simulink model "PFMS_Aerosonde_Model"  (Simulink 7.3)
settings: Solver=ode4  SolverMode=SingleTasking  StartTime=0.0  StopTime=inf  FixedStep=0.008  RelTol=1e-3
undefined symbols (not defined in the file or in its folder): b, heading, J, waypoint
libraries: aerosimlib x29, simulink_extras x5
CloseFcn:
  | rtwprivate ssgencode ModelCloseRequest PFMS
settings Model: Creator=Nicholas  LastModifiedBy=user
settings DataIOCC: LimitDataPoints=off  SaveOutput=off  SaveTime=off
settings OptimizationCC: BlockReduction=off  BooleanDataType=off
settings DebuggingCC: SaveWithParameterizedLinksMsg=none  SignalResolutionControl=TryResolveAllWithWarning  SolverPrmCheckMsg=none  MultiTaskDSMMsg=warning  MultiTaskCondExecSysMsg=none  UnconnectedInputMsg=none  UnconnectedOutputMsg=none  UnconnectedLineMsg=none  StrictBusMsg=None
settings HardwareCC: TargetEndianess=LittleEndian  TargetHWDeviceType=MATLAB Host  ProdEqTarget=off
settings RTWCC: IncludeERTFirstTime=on

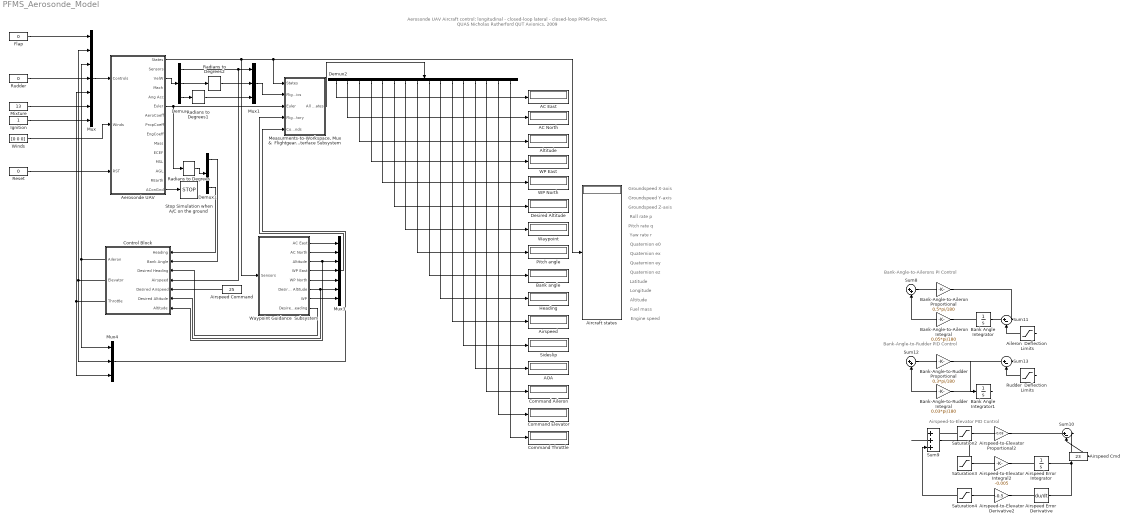
== system PFMS_Aerosonde_Model ==
  note: Groundspeed X-axis
  note: Groundspeed Y-axis
  note: Groundspeed Z-axis
  note: Roll rate p
  note: Pitch rate q
  note: Yaw rate r
  note: Quaternion e0
  note: Quaternion ex
  note: Quaternion ey
  note: Quaternion ez
  note: Latitude
  note: Longitude
  note: Altitude
  note: Fuel mass
  note: Engine speed
  note: Aerosonde UAV
      | Aircraft control: longitudinal - closed-loop
      |   lateral - closed-loop
      | PFMS Project, QUAS
      | Nicholas Rutherford
      | QUT Avionics, 2009
  note: Bank-Angle-to-Ailerons PI Control
  note: Airspeed-to-Elevator PID Control
  note: Bank-Angle-to-Rudder PID Control
  AC East : Display
  AC North : Display
  AOA : Display
  Aerosonde UAV : Subsystem  mask(6-DOF Aircraft Model){aircraftcfg='aerosondecfg.mat', VelocitiesIni=[23 0 0]', RatesIni=[0 0 0]', QuaternionsIni=[1 0 0 0]', PositionIni=[-0.4877  2.6728 1000]', FuelIni=2, OmegaIni=5000*pi/30, GndAlt=20, wmmfile='C:\Program Files\MATLAB\AeroSim\wmm.cof', dmy=[26 05 2009], tsamp=0.8}
      mask prompts: aircraftcfg "Aircraft configuration file:"; VelocitiesIni "Initial velocities:"; RatesIni "Initial angular rates:"; QuaternionsIni "Initial attitude:"; PositionIni "Initial position:"; FuelIni "Initial fuel mass:"; OmegaIni "Initial engine speed:"; GndAlt "Ground altitude:"; wmmfile "WMM coefficient file:"; dmy "Simulation date:"; tsamp "Sample time:"
      mask help: Nonlinear 6-DOF aircraft model with equations of motion in body frame.
      mask init:
      | load(aircraftcfg);
      mask Help:
      | The block implements the 6-DOF nonlinear aircraft model using AeroSim blocks. Velocities are computed in body frame.
      | <P><B>Inputs:</B>
      | <LI>Controls = the 7x1 vector of aircraft controls [flap elevator aileron rudder throttle mixture ignition]. Aerodynamic controls are in radians, throttle is from 0 to 1, mixture is fraction air/fuel flow, ignition is 0 (engine off) or 1 (engine on).</LI>
      | <LI>Winds = the 3x1 vector of background wind speed components in navigation frame [North East Down]</LI>
      | <LI>RST = the integrator reset flag (0 or 1, all integrators on rising edge)
      | </P>
      | <P><B>Outputs:</B>
      | <LI>States = the 15x1 aircraft state vector [Velocities, Angular rates, Quaternions, Position, Fuel mass, Engine speed].</LI>
      | <LI>Sensors = the 18x1 vector of sensor outputs [GPS Position, GPS Groundspeed, Accelerometers, Gyros, Air data, Magnetometer].</LI>
      | <LI>VelW = the 3x1 vector of aircraft velocity in wind axes [Airspeed, sideslip, angle of attack]</LI>
      | <LI>Mach = the Mach number</LI>
      | <LI>Ang Acc = the 3x1 vector of angular accelerations
      | <LI>Euler = the 3x1 vector of Euler angles (roll, pitch, yaw)</LI>
      | <LI>AeroCoeff = the 6x1 vector of aerodynamic coefficients [CD CY CL Cl Cm Cn]</LI>
      | <LI>PropCoeff = the 3x1 vector of propeller coefficients [J CT CP]</LI>
      | <LI>EngCoeff = the 5x1 vector of engine coefficients [MAP Airflow Fuelflow BSFC Power]</LI>
      | <LI>Mass = the current aircraft mass</LI>
      | <LI>ECEF = 3x1 vector of position of the aircraft in the Earth-centered, Earth-fixed frame</LI>
      | <LI>MSL = the aircraft altitude above mean-sea-level</LI>
      | <LI>AGL = the aircraft altitude above terrain</LI>
      | <LI>REarth = the Earth equivalent radius at current location
      | <LI>AConGnd = the aircraft-on-ground flag (0 if aircraft above ground, 1 if aircraft on the ground)</LI>
      | </P>
      | <P><B>Parameters:</B>
      | <LI>Aircraft configuration file = the MAT-file with aircraft data</LI>
      | <LI>Initial velocities = the 3x1 vector of initial aircraft velocities in body axes [u v w]</LI>
      | <LI>Initial angular rates = the 3x1 vector of initial angular rates [p q r]</LI>
      | <LI>Initial attitude = the 4x1 vector of initial quaternions [e0 ex ey ez]</LI>
      | <LI>Initial position = the 3x1 vector of initial aircraft location [Lat Lon Alt]</LI>
      | <LI>Initial fuel mass = the initial quantity of fuel on-board the aircraft</LI>
      | <LI>Initial engine speed = the initial engine rotation speed</LI>
      | <LI>Ground altitude = the ground altitude at aircraft location</LI>
      | <LI>WMM coefficient file = the path to the magnetic model coefficient file</LI>
      | <LI>Simulation date = the date to be used for the magnetic model [day month year]</LI>
      | <LI>Sample time = the aircraft model sample time.</LI>
      | </P>
  Aileron  Deflection  Limits : Saturate  UpperLimit=+20  LowerLimit=-20
  Aircraft states : Display
  Airspeed : Display
  Airspeed Cmd : Constant  Value=23  OutDataType=sfix(16)  OutScaling=2^0
  Airspeed Command : Constant  Value=25
  Airspeed Error Derivative : Derivative
  Airspeed Error Integrator : Integrator
  Airspeed-to-Elevator Derivative2 : Gain  Gain=-0.5  ParameterDataType=sfix(16)  ParameterScaling=2^0  OutDataType=sfix(16)  OutScaling=2^0  SaturateOnIntegerOverflow=on  OutDataTypeStr=Inherit: Same as input  ParamDataTypeStr=Inherit: Same as input
  Airspeed-to-Elevator Integral2 : Gain  Gain=-0.005  ParameterDataType=sfix(16)  ParameterScaling=2^0  OutDataType=sfix(16)  OutScaling=2^0  SaturateOnIntegerOverflow=on  OutDataTypeStr=Inherit: Same as input  ParamDataTypeStr=Inherit: Same as input
  Airspeed-to-Elevator Proportional2 : Gain  Gain=-0.03  ParameterDataType=sfix(16)  ParameterScaling=2^0  OutDataType=sfix(16)  OutScaling=2^0  SaturateOnIntegerOverflow=on  OutDataTypeStr=Inherit: Same as input  ParamDataTypeStr=Inherit: Same as input
  Altitude : Display
  Bank Angle Integrator : Integrator
  Bank Angle Integrator1 : Integrator
  Bank angle : Display
  Bank-Angle-to-Aileron Integral : Gain  Gain=0.05*pi/180  ParameterDataType=sfix(16)  ParameterScaling=2^0  OutDataType=sfix(16)  OutScaling=2^0  SaturateOnIntegerOverflow=on  OutDataTypeStr=Inherit: Same as input  ParamDataTypeStr=Inherit: Same as input
  Bank-Angle-to-Aileron Proportional : Gain  Gain=0.5*pi/180  ParameterDataType=sfix(16)  ParameterScaling=2^0  OutDataType=sfix(16)  OutScaling=2^0  SaturateOnIntegerOverflow=on  OutDataTypeStr=Inherit: Same as input  ParamDataTypeStr=Inherit: Same as input
  Bank-Angle-to-Rudder Integral : Gain  Gain=0.03*pi/180  ParameterDataType=sfix(16)  ParameterScaling=2^0  OutDataType=sfix(16)  OutScaling=2^0  SaturateOnIntegerOverflow=on  OutDataTypeStr=Inherit: Same as input  ParamDataTypeStr=Inherit: Same as input
  Bank-Angle-to-Rudder Proportional : Gain  Gain=0.3*pi/180  ParameterDataType=sfix(16)  ParameterScaling=2^0  OutDataType=sfix(16)  OutScaling=2^0  SaturateOnIntegerOverflow=on  OutDataTypeStr=Inherit: Same as input  ParamDataTypeStr=Inherit: Same as input
  Command Aileron : Display
  Command Elevator : Display
  Command Throttle : Display
  Control Block : Subsystem
  Demux : Demux  Outputs=3
  Demux1 : Demux  Outputs=3
  Demux2 : Demux  Outputs=16
  Desired Altitude : Display
  Flap : Constant  Value=0
  Heading : Display
  Ignition : Constant
  "Measurments-to-Workspace, Mux &  Flightgear Interface Subsystem" : Subsystem
  Mixture : Constant  Value=13
  Mux : Mux  Inputs=7
  Mux1 : Mux  Inputs=3
  Mux3 : Mux  Inputs=7
  Mux4 : Mux  Inputs=3
  Pitch angle : Display
  Radians to Degrees : simulink_extras/Transformations/Radians to Degrees  SystemSampleTime=-1
  Radians to Degrees1 : simulink_extras/Transformations/Radians to Degrees  SystemSampleTime=-1
  Radians to Degrees2 : simulink_extras/Transformations/Radians to Degrees  SystemSampleTime=-1
  Reset : Constant  Value=0
  Rudder : Constant  Value=0
  Rudder  Deflection  Limits : Saturate  UpperLimit=+15  LowerLimit=-15
  Saturation2 : Saturate  UpperLimit=+5  LowerLimit=-5
  Saturation3 : Saturate  UpperLimit=+10  LowerLimit=-10
  Saturation4 : Saturate  UpperLimit=+5  LowerLimit=-5
  Sideslip : Display
  Stop Simulation when A/C on the ground : Stop
  Sum10 : Sum  Inputs=|+-  OutDataType=sfix(16)  OutScaling=2^0  SaturateOnIntegerOverflow=on  InputSameDT=on  OutDataTypeStr=Inherit: Same as first input
  Sum11 : Sum  Inputs=|+-  OutDataType=sfix(16)  OutScaling=2^0  SaturateOnIntegerOverflow=on  InputSameDT=on  OutDataTypeStr=Inherit: Same as first input
  Sum12 : Sum  Inputs=|++  OutDataType=sfix(16)  OutScaling=2^0  SaturateOnIntegerOverflow=on  InputSameDT=on  OutDataTypeStr=Inherit: Same as first input
  Sum13 : Sum  Inputs=|+-  OutDataType=sfix(16)  OutScaling=2^0  SaturateOnIntegerOverflow=on  InputSameDT=on  OutDataTypeStr=Inherit: Same as first input
  Sum8 : Sum  Inputs=|++  OutDataType=sfix(16)  OutScaling=2^0  SaturateOnIntegerOverflow=on  InputSameDT=on  OutDataTypeStr=Inherit: Same as first input
  Sum9 : Sum  Inputs=+++  OutDataType=sfix(16)  OutScaling=2^0  SaturateOnIntegerOverflow=on  InputSameDT=on  OutDataTypeStr=Inherit: Same as first input
  WP East : Display
  WP North : Display
  Waypoint : Display
  Waypoint Guidance  Subsystem : Subsystem
  Winds : Constant  Value=[0 0 0]
  wires:
  Reset/1 -> Aerosonde UAV/3(RST)
  Winds/1 -> Aerosonde UAV/2(Winds)
  Aerosonde UAV/1(States) -> Waypoint Guidance  Subsystem/1(Sensors), Aircraft states/1, "Measurments-to-Workspace, Mux &  Flightgear Interface Subsystem"/1(States)
  Aerosonde UAV/6(Euler) -> Radians to Degrees/1, "Measurments-to-Workspace, Mux &  Flightgear Interface Subsystem"/3(Euler)
  Aerosonde UAV/3(VelW) -> Demux/1
  Demux/3 -> Radians to Degrees1/1
  Demux/2 -> Radians to Degrees2/1
  Demux/1 -> Control Block/4(Airspeed), Mux1/1
  Aerosonde UAV/15(AConGnd) -> Stop Simulation when A/C on the ground/1
  Radians to Degrees/1 -> Demux1/1
  Demux1/1 -> Control Block/2(Bank Angle)
  Rudder/1 -> Mux/4
  Mixture/1 -> Mux/6
  Demux1/3 -> Control Block/1(Heading)
  Airspeed Command/1 -> Control Block/5(Desired Airspeed)
  ? -> Sum13/1, Sum11/1
  Bank-Angle-to-Aileron Proportional/1 -> Sum8/1
  Bank Angle Integrator/1 -> Bank-Angle-to-Aileron Integral/1
  Bank-Angle-to-Aileron Integral/1 -> Sum8/2
  Airspeed Error Derivative/1 -> Airspeed-to-Elevator Derivative2/1
  Airspeed Error Integrator/1 -> Airspeed-to-Elevator Integral2/1
  Airspeed-to-Elevator Proportional2/1 -> Saturation2/1
  Airspeed-to-Elevator Integral2/1 -> Saturation3/1
  Airspeed-to-Elevator Derivative2/1 -> Saturation4/1
  Sum10/1 -> Airspeed-to-Elevator Proportional2/1, Airspeed Error Integrator/1, Airspeed Error Derivative/1
  Sum11/1 -> Bank-Angle-to-Aileron Proportional/1, Bank Angle Integrator/1
  Bank-Angle-to-Rudder Proportional/1 -> Sum12/1
  Bank Angle Integrator1/1 -> Bank-Angle-to-Rudder Integral/1
  Bank-Angle-to-Rudder Integral/1 -> Sum12/2
  Sum13/1 -> Bank-Angle-to-Rudder Proportional/1, Bank Angle Integrator1/1
  Rudder  Deflection  Limits/1 -> Sum13/2
  Aileron  Deflection  Limits/1 -> Sum11/2
  Airspeed Cmd/1 -> Sum10/2
  ? -> Rudder  Deflection  Limits/1, Aileron  Deflection  Limits/1
  Saturation2/1 -> Sum9/1
  Saturation3/1 -> Sum9/2
  Saturation4/1 -> Sum9/3
  ? -> Sum10/1
  Sum8/1 -> ?
  Sum12/1 -> ?
  Sum9/1 -> ?
  Flap/1 -> Mux/1
  Ignition/1 -> Mux/7
  Mux/1 -> Aerosonde UAV/1(Controls)
  Waypoint Guidance  Subsystem/2(AC North) -> Mux3/2
  Waypoint Guidance  Subsystem/4(WP East) -> Mux3/4
  Waypoint Guidance  Subsystem/5(WP North) -> Mux3/5
  Waypoint Guidance  Subsystem/3(Altitude) -> Mux3/3, Control Block/7(Altitude)
  Waypoint Guidance  Subsystem/6(Desired Altitude) -> Mux3/6, Control Block/6(Desired Altitude)
  Waypoint Guidance  Subsystem/8(Desired Heading) -> Control Block/3(Desired Heading)
  Radians to Degrees2/1 -> Mux1/2
  Radians to Degrees1/1 -> Mux1/3
  Mux1/1 -> "Measurments-to-Workspace, Mux &  Flightgear Interface Subsystem"/2(Flight Dynamics)
  Mux3/1 -> "Measurments-to-Workspace, Mux &  Flightgear Interface Subsystem"/4(Flight Trajectory)
  Mux4/1 -> "Measurments-to-Workspace, Mux &  Flightgear Interface Subsystem"/5(Control Commands)
  "Measurments-to-Workspace, Mux &  Flightgear Interface Subsystem"/1(All States) -> Demux2/1
  Waypoint Guidance  Subsystem/7(WP) -> Mux3/7
  Waypoint Guidance  Subsystem/1(AC East) -> Mux3/1
  Control Block/1(Aileron) -> Mux/3, Mux4/1
  Control Block/2(Elevator) -> Mux/2, Mux4/2
  Control Block/3(Throttle) -> Mux4/3, Mux/5
  Demux2/1 -> AC East/1
  Demux2/2 -> AC North/1
  Demux2/3 -> Altitude/1
  Demux2/4 -> WP East/1
  Demux2/5 -> WP North/1
  Demux2/6 -> Desired Altitude/1
  Demux2/7 -> Waypoint/1
  Demux2/8 -> Pitch angle/1
  Demux2/9 -> Bank angle/1
  Demux2/10 -> Heading/1
  Demux2/11 -> Airspeed/1
  Demux2/12 -> Sideslip/1
  Demux2/13 -> AOA/1
  Demux2/14 -> Command Aileron/1
  Demux2/15 -> Command Elevator/1
  Demux2/16 -> Command Throttle/1

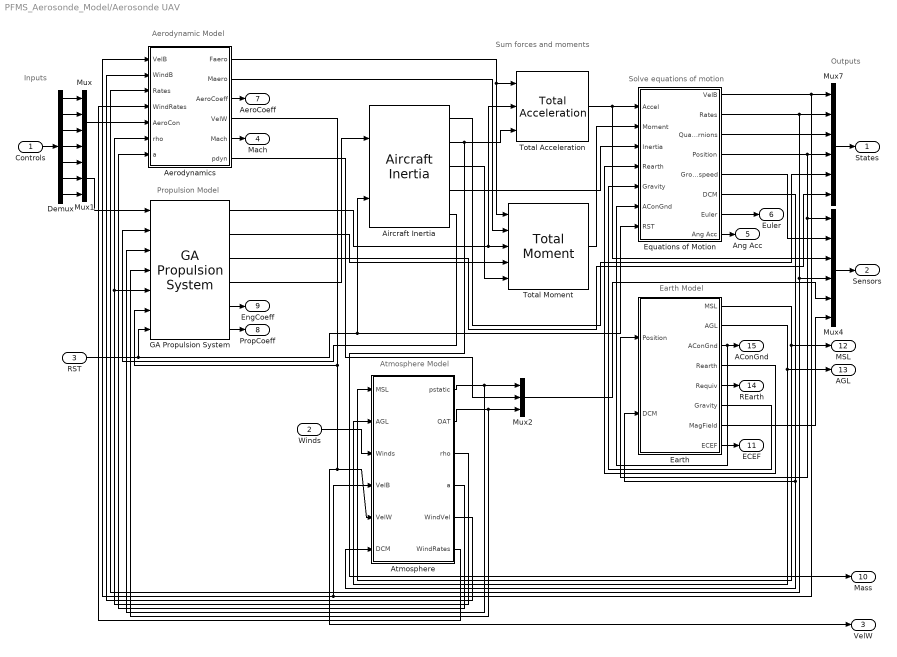
== system PFMS_Aerosonde_Model/Aerosonde UAV ==
  note: Solve equations of motion
  note: Inputs
  note: Outputs
  note: Aerodynamic Model
  note: Earth Model
  note: Sum forces and moments
  note: Atmosphere Model
  note: Propulsion Model
  Controls : Inport  OutDataType=sfix(16)  OutScaling=2^0
  Winds : Inport  Port=2  OutDataType=sfix(16)  OutScaling=2^0
  RST : Inport  Port=3  OutDataType=sfix(16)  OutScaling=2^0
  Aerodynamics : Subsystem
  Aircraft Inertia : aerosimlib/Inertia/Aircraft Inertia  SystemSampleTime=-1  FuelIni=FuelIni  Mempty=mempty  Mgross=mgross  CGempty=CGempty  CGgross=CGgross  Jempty=Jempty  Jgross=Jgross
  Atmosphere : Subsystem
  Demux : Demux  Outputs=7
  Earth : Subsystem
  Equations of Motion : Subsystem
  GA Propulsion System : aerosimlib/Propulsion/GA Propulsion System  SystemSampleTime=-1  OmegaIni=OmegaIni  RPM=RPM  MAP=MAP  FuelFlow=FuelFlow  Power=Power  Jeng=Jeng  J=J  CT=CT  CP=CP  Rprop=Rprop  Jprop=Jprop  TSL=TSL
  Mux : Mux
  Mux1 : Mux  Inputs=3
  Mux2 : Mux  Inputs=3
  Mux4 : Mux  Inputs=6
  Mux7 : Mux  Inputs=6
  Total Acceleration : aerosimlib/Equations of Motion/Total Acceleration  SystemSampleTime=-1
  Total Moment : aerosimlib/Equations of Motion/Total Moment  SystemSampleTime=-1  raero=rAC  rprop=rHub
  States : Outport
  Sensors : Outport  Port=2
  VelW : Outport  Port=3
  Mach : Outport  Port=4
  Ang Acc : Outport  Port=5
  Euler : Outport  Port=6
  AeroCoeff : Outport  Port=7
  PropCoeff : Outport  Port=8
  EngCoeff : Outport  Port=9
  Mass : Outport  Port=10
  ECEF : Outport  Port=11
  MSL : Outport  Port=12
  AGL : Outport  Port=13
  REarth : Outport  Port=14
  AConGnd : Outport  Port=15
  wires:
  Equations of Motion/7(Euler) -> Euler/1
  Equations of Motion/8(Ang Acc) -> Ang Acc/1
  Atmosphere/6(WindRates) -> Aerodynamics/4(WindRates)
  RST/1 -> Aircraft Inertia/2, Equations of Motion/7(RST), GA Propulsion System/7
  Aircraft Inertia/5 -> GA Propulsion System/2
  Atmosphere/4(a) -> Aerodynamics/7(a)
  Atmosphere/3(rho) -> GA Propulsion System/5, Aerodynamics/6(rho)
  Atmosphere/5(WindVel) -> Aerodynamics/2(WindB)
  Winds/1 -> Atmosphere/3(Winds)
  Earth/2(AGL) -> AGL/1, Atmosphere/2(AGL)
  Earth/1(MSL) -> MSL/1, Atmosphere/1(MSL)
  Aerodynamics/4(VelW) -> VelW/1, Atmosphere/5(VelW), GA Propulsion System/6
  GA Propulsion System/4 -> Aircraft Inertia/1
  GA Propulsion System/3 -> Mux7/6
  Aircraft Inertia/1 -> Mux7/5
  Mux2/1 -> Mux4/5
  Aerodynamics/6(pdyn) -> Mux2/2
  Atmosphere/2(OAT) -> GA Propulsion System/4, Mux2/3
  Atmosphere/1(pstatic) -> GA Propulsion System/3, Mux2/1
  Equations of Motion/6(DCM) -> Atmosphere/6(DCM), Earth/2(DCM)
  GA Propulsion System/2 -> Total Moment/4
  GA Propulsion System/1 -> Total Moment/3, Total Acceleration/2
  Aerodynamics/2(Maero) -> Total Moment/2
  Aerodynamics/1(Faero) -> Total Moment/1, Total Acceleration/1
  Aircraft Inertia/3 -> Total Moment/5
  Total Moment/1 -> Equations of Motion/2(Moment)
  Aircraft Inertia/4 -> Equations of Motion/3(Inertia)
  Aircraft Inertia/2 -> Mass/1, Total Acceleration/3
  Earth/4(Rearth) -> Equations of Motion/4(Rearth)
  Earth/6(Gravity) -> Equations of Motion/5(Gravity)
  Earth/7(MagField) -> Mux4/6
  Total Acceleration/1 -> Mux4/3, Equations of Motion/1(Accel)
  Equations of Motion/5(Groundspeed) -> Mux4/2
  Earth/3(AConGnd) -> Equations of Motion/6(AConGnd), AConGnd/1
  Earth/5(Requiv) -> REarth/1
  GA Propulsion System/6 -> PropCoeff/1
  GA Propulsion System/5 -> EngCoeff/1
  Demux/7 -> Mux1/3
  Demux/6 -> Mux1/2
  Demux/5 -> Mux1/1
  Demux/4 -> Mux/4
  Demux/3 -> Mux/3
  Demux/2 -> Mux/2
  Demux/1 -> Mux/1
  Controls/1 -> Demux/1
  Mux4/1 -> Sensors/1
  Mux7/1 -> States/1
  Mux1/1 -> GA Propulsion System/1
  Equations of Motion/1(VelB) -> Aerodynamics/1(VelB), Atmosphere/4(VelB), Mux7/1
  Equations of Motion/2(Rates) -> Aerodynamics/3(Rates), Mux4/4, Mux7/2
  Equations of Motion/4(Position) -> Earth/1(Position), Mux4/1, Mux7/4
  Mux/1 -> Aerodynamics/5(AeroCon)
  Equations of Motion/3(Quaternions) -> Mux7/3
  Aerodynamics/5(Mach) -> Mach/1
  Aerodynamics/3(AeroCoeff) -> AeroCoeff/1
  Earth/8(ECEF) -> ECEF/1

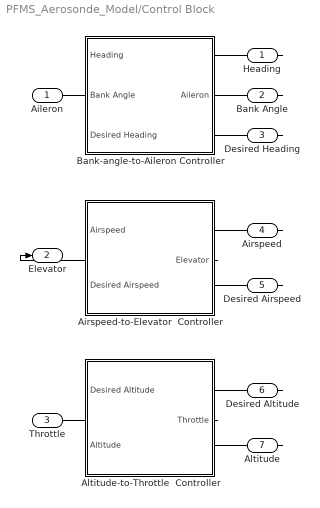
== system PFMS_Aerosonde_Model/Control Block ==
  Heading : Inport
  Bank Angle : Inport  Port=2
  Desired Heading : Inport  Port=3
  Airspeed : Inport  Port=4
  Desired Airspeed : Inport  Port=5
  Desired Altitude : Inport  Port=6
  Altitude : Inport  Port=7
  Airspeed-to-Elevator  Controller : Subsystem
  Altitude-to-Throttle  Controller : Subsystem
  Bank-angle-to-Aileron Controller : Subsystem
  Aileron : Outport
  Elevator : Outport  Port=2
  Throttle : Outport  Port=3
  wires:
  Heading/1 -> Bank-angle-to-Aileron Controller/1(Heading)
  Bank Angle/1 -> Bank-angle-to-Aileron Controller/2(Bank Angle)
  Bank-angle-to-Aileron Controller/1(Aileron) -> Aileron/1
  Desired Heading/1 -> Bank-angle-to-Aileron Controller/3(Desired Heading)
  Airspeed/1 -> Airspeed-to-Elevator  Controller/1(Airspeed)
  Airspeed-to-Elevator  Controller/1(Elevator) -> Elevator/1
  Desired Airspeed/1 -> Airspeed-to-Elevator  Controller/2(Desired Airspeed)
  Desired Altitude/1 -> Altitude-to-Throttle  Controller/1(Desired Altitude)
  Altitude-to-Throttle  Controller/1(Throttle) -> Throttle/1
  Altitude/1 -> Altitude-to-Throttle  Controller/2(Altitude)

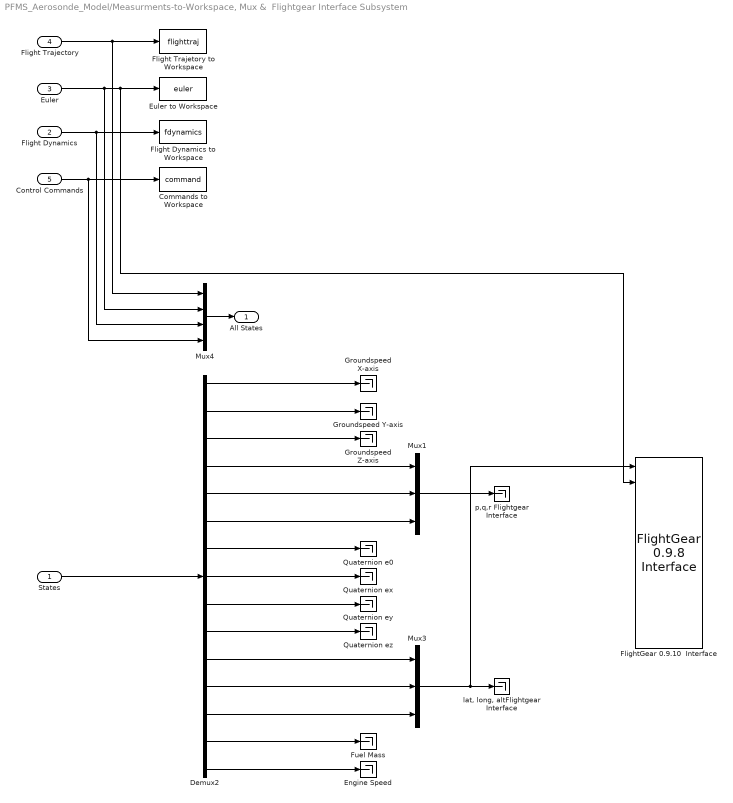
== system PFMS_Aerosonde_Model/Measurments-to-Workspace, Mux &  Flightgear Interface Subsystem ==
  States : Inport
  Flight Dynamics : Inport  Port=2
  Euler : Inport  Port=3
  Flight Trajectory : Inport  Port=4
  Control Commands : Inport  Port=5
  Commands to Workspace : ToWorkspace  VariableName=command  SampleTime=-1  SaveFormat=Structure
  Demux2 : Demux  Outputs=15
  Engine Speed : Terminator
  Euler to Workspace : ToWorkspace  VariableName=euler  SampleTime=-1  SaveFormat=Structure
  Flight Dynamics to Workspace : ToWorkspace  VariableName=fdynamics  SampleTime=-1  SaveFormat=Structure
  Flight Trajetory to Workspace : ToWorkspace  VariableName=flighttraj  SampleTime=-1  SaveFormat=Structure
  FlightGear 0.9.10  Interface : aerosimlib/Pilot Interface/FlightGear 0.9.8  Interface  SystemSampleTime=-1  hostname='localhost'  port=5500  tsamp=0.04
      link override S-Function: FunctionName=sfunflightgear0910
  Fuel Mass : Terminator
  Groundspeed X-axis : Terminator
  Groundspeed Y-axis : Terminator
  Groundspeed Z-axis : Terminator
  Mux1 : Mux  Inputs=3
  Mux3 : Mux  Inputs=3
  Mux4 : Mux
  Quaternion e0 : Terminator
  Quaternion ex : Terminator
  Quaternion ey : Terminator
  Quaternion ez : Terminator
  "lat, long, altFlightgear Interface" : Terminator
  p,q,r Flightgear Interface : Terminator
  All States : Outport  OutDataType=fixdt(1, 16)  OutScaling=2^0
  wires:
  Euler/1 -> Mux4/2, Euler to Workspace/1, FlightGear 0.9.10  Interface/2
  Flight Trajectory/1 -> Flight Trajetory to Workspace/1, Mux4/1
  Flight Dynamics/1 -> Flight Dynamics to Workspace/1, Mux4/3
  Control Commands/1 -> Commands to Workspace/1, Mux4/4
  Mux4/1 -> All States/1
  Demux2/1 -> Groundspeed X-axis/1
  Demux2/2 -> Groundspeed Y-axis/1
  Demux2/3 -> Groundspeed Z-axis/1
  Demux2/4 -> Mux1/1
  Demux2/8 -> Quaternion ex/1
  Demux2/9 -> Quaternion ey/1
  Demux2/10 -> Quaternion ez/1
  Demux2/14 -> Fuel Mass/1
  Demux2/15 -> Engine Speed/1
  Demux2/11 -> Mux3/1
  Demux2/12 -> Mux3/2
  Demux2/13 -> Mux3/3
  States/1 -> Demux2/1
  Demux2/5 -> Mux1/2
  Demux2/6 -> Mux1/3
  Demux2/7 -> Quaternion e0/1
  Mux1/1 -> p,q,r Flightgear Interface/1
  Mux3/1 -> "lat, long, altFlightgear Interface"/1, FlightGear 0.9.10  Interface/1

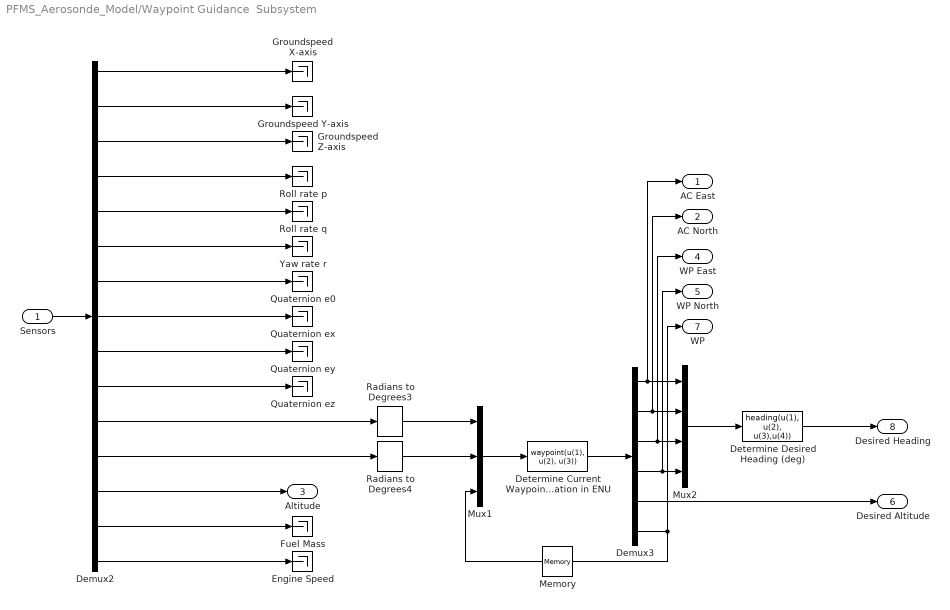
== system PFMS_Aerosonde_Model/Waypoint Guidance  Subsystem ==
  Sensors : Inport
  Demux2 : Demux  Outputs=15
  Demux3 : Demux  Outputs=6
  Determine Current Waypoint & A/C Location in ENU : MATLABFcn  MATLABFcn=waypoint(u(1), u(2), u(3))  OutputDimensions=6
  Determine Desired Heading (deg) : MATLABFcn  MATLABFcn=heading(u(1), u(2), u(3),u(4))  OutputDimensions=1
  Engine Speed : Terminator
  Fuel Mass : Terminator
  Groundspeed X-axis : Terminator
  Groundspeed Y-axis : Terminator
  Groundspeed Z-axis : Terminator
  Memory : Memory  X0=1
  Mux1 : Mux  Inputs=3
  Mux2 : Mux
  Quaternion e0 : Terminator
  Quaternion ex : Terminator
  Quaternion ey : Terminator
  Quaternion ez : Terminator
  Radians to Degrees3 : simulink_extras/Transformations/Radians to Degrees  SystemSampleTime=-1
  Radians to Degrees4 : simulink_extras/Transformations/Radians to Degrees  SystemSampleTime=-1
  Roll rate p : Terminator
  Roll rate q : Terminator
  Yaw rate r : Terminator
  AC East : Outport
  AC North : Outport  Port=2
  Altitude : Outport  Port=3
  WP East : Outport  Port=4
  WP North : Outport  Port=5
  Desired Altitude : Outport  Port=6
  WP : Outport  Port=7
  Desired Heading : Outport  Port=8
  wires:
  Mux1/1 -> Determine Current Waypoint & A/C Location in ENU/1
  Memory/1 -> Mux1/3
  Determine Current Waypoint & A/C Location in ENU/1 -> Demux3/1
  Demux3/1 -> Mux2/1, AC East/1
  Demux3/3 -> Mux2/3, WP East/1
  Demux3/4 -> Mux2/4, WP North/1
  Mux2/1 -> Determine Desired Heading (deg)/1
  Demux2/11 -> Radians to Degrees3/1
  Radians to Degrees3/1 -> Mux1/1
  Demux2/12 -> Radians to Degrees4/1
  Radians to Degrees4/1 -> Mux1/2
  Demux3/2 -> Mux2/2, AC North/1
  Demux3/6 -> Memory/1, WP/1
  Demux2/1 -> Groundspeed X-axis/1
  Demux2/2 -> Groundspeed Y-axis/1
  Demux2/3 -> Groundspeed Z-axis/1
  Demux2/4 -> Roll rate p/1
  Demux2/5 -> Roll rate q/1
  Demux2/6 -> Yaw rate r/1
  Demux2/7 -> Quaternion e0/1
  Demux2/8 -> Quaternion ex/1
  Demux2/9 -> Quaternion ey/1
  Demux2/10 -> Quaternion ez/1
  Demux2/14 -> Fuel Mass/1
  Demux2/15 -> Engine Speed/1
  Sensors/1 -> Demux2/1
  Determine Desired Heading (deg)/1 -> Desired Heading/1
  Demux2/13 -> Altitude/1
  Demux3/5 -> Desired Altitude/1

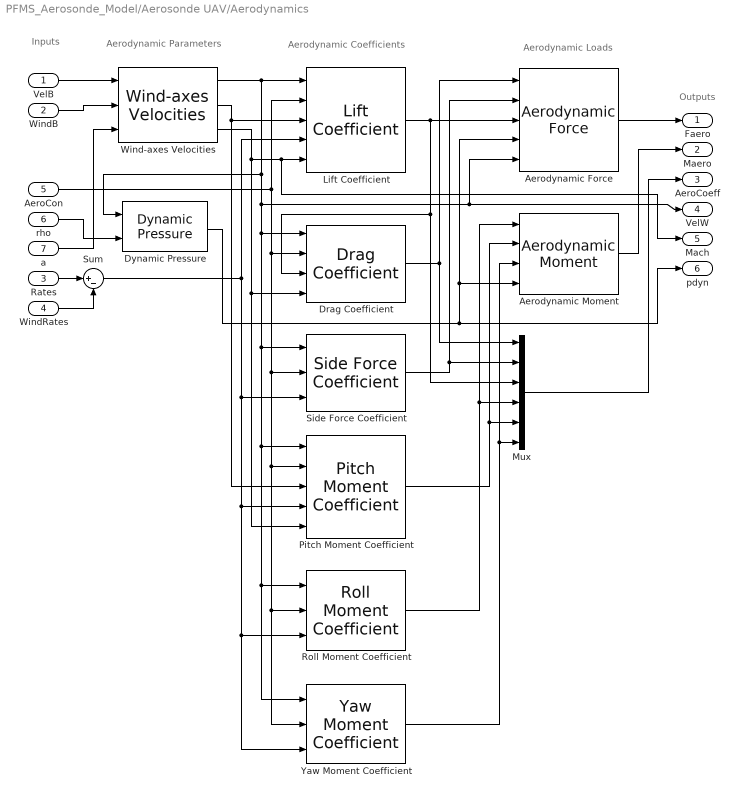
== system PFMS_Aerosonde_Model/Aerosonde UAV/Aerodynamics ==
  note: Inputs
  note: Outputs
  note: Aerodynamic Parameters
  note: Aerodynamic Coefficients
  note: Aerodynamic Loads
  VelB : Inport  PortDimensions=[3 1]  OutDataType=sfix(16)  OutScaling=2^0
  WindB : Inport  Port=2  PortDimensions=[3 1]  OutDataType=sfix(16)  OutScaling=2^0
  Rates : Inport  Port=3  PortDimensions=[3 1]  OutDataType=sfix(16)  OutScaling=2^0
  WindRates : Inport  Port=4  PortDimensions=[3 1]  OutDataType=sfix(16)  OutScaling=2^0
  AeroCon : Inport  Port=5  PortDimensions=[4 1]  OutDataType=sfix(16)  OutScaling=2^0
  rho : Inport  Port=6  PortDimensions=1  OutDataType=sfix(16)  OutScaling=2^0
  a : Inport  Port=7  PortDimensions=1  OutDataType=sfix(16)  OutScaling=2^0
  Aerodynamic Force : aerosimlib/Aerodynamics/Aerodynamic Force  SystemSampleTime=-1  S=S
  Aerodynamic Moment : aerosimlib/Aerodynamics/Aerodynamic Moment  SystemSampleTime=-1  c=MAC  b=b  S=S
  Drag Coefficient : aerosimlib/Aerodynamics/Drag Coefficient  SystemSampleTime=-1  CL0=CLmind  CD0=CDmin  CDdf=CDdf  CDde=CDde  CDda=CDda  CDdr=CDdr  CDM=CDM  e=osw  b=b  S=S
  Dynamic Pressure : aerosimlib/Aerodynamics/Dynamic Pressure  SystemSampleTime=-1
  Lift Coefficient : aerosimlib/Aerodynamics/Lift Coefficient  SystemSampleTime=-1  CL0=CL0  CLalpha=CLa  CLdf=CLdf  CLde=CLde  CLalphadot=CLalphadot  CLq=CLq  CLM=CLM  c=MAC
  Mux : Mux  Inputs=6
  Pitch Moment Coefficient : aerosimlib/Aerodynamics/Pitch Moment Coefficient  SystemSampleTime=-1  Cm0=Cm0  Cma=Cma  Cmdf=Cmdf  Cmde=Cmde  Cmalphadot=Cmalphadot  Cmq=Cmq  CmM=CmM  c=MAC
  Roll Moment Coefficient : aerosimlib/Aerodynamics/Roll Moment Coefficient  SystemSampleTime=-1  Clbeta=Clbeta  Clda=Clda  Cldr=Cldr  Clp=Clp  Clr=Clr  b=b
  Side Force Coefficient : aerosimlib/Aerodynamics/Side Force Coefficient  SystemSampleTime=-1  CYbeta=CYbeta  CYda=CYda  CYdr=CYdr  CYp=CYp  CYr=CYr  b=b
  Sum : Sum  Inputs=|+-  OutDataType=sfix(16)  OutScaling=2^0  SaturateOnIntegerOverflow=on  InputSameDT=on  OutDataTypeStr=Inherit: Same as first input
  Wind-axes Velocities : aerosimlib/Aerodynamics/Wind-axes Velocities  SystemSampleTime=-1  Vabnd=VaBnd  betabnd=BetaBnd  alphabnd=AlphaBnd
  Yaw Moment Coefficient : aerosimlib/Aerodynamics/Yaw Moment Coefficient  SystemSampleTime=-1  Cnbeta=Cnbeta  Cnda=Cnda  Cndr=Cndr  Cnp=Cnp  Cnr=Cnr  b=b
  Faero : Outport
  Maero : Outport  Port=2
  AeroCoeff : Outport  Port=3
  VelW : Outport  Port=4
  Mach : Outport  Port=5
  pdyn : Outport  Port=6
  wires:
  Sum/1 -> Roll Moment Coefficient/3, Yaw Moment Coefficient/3, Pitch Moment Coefficient/4, Side Force Coefficient/3, Lift Coefficient/4
  WindRates/1 -> Sum/2
  Rates/1 -> Sum/1
  Mux/1 -> AeroCoeff/1
  Aerodynamic Moment/1 -> Maero/1
  Aerodynamic Force/1 -> Faero/1
  Yaw Moment Coefficient/1 -> Mux/6, Aerodynamic Moment/3
  Pitch Moment Coefficient/1 -> Mux/5, Aerodynamic Moment/2
  Roll Moment Coefficient/1 -> Mux/4, Aerodynamic Moment/1
  Dynamic Pressure/1 -> pdyn/1, Aerodynamic Moment/4, Aerodynamic Force/4
  Side Force Coefficient/1 -> Mux/2, Aerodynamic Force/2
  Drag Coefficient/1 -> Mux/1, Aerodynamic Force/1
  Lift Coefficient/1 -> Mux/3, Drag Coefficient/3, Aerodynamic Force/3
  Wind-axes Velocities/3 -> Mach/1, Lift Coefficient/5, Pitch Moment Coefficient/5, Drag Coefficient/4
  Wind-axes Velocities/2 -> Pitch Moment Coefficient/3, Lift Coefficient/3
  AeroCon/1 -> Yaw Moment Coefficient/2, Roll Moment Coefficient/2, Pitch Moment Coefficient/2, Side Force Coefficient/2, Drag Coefficient/2, Lift Coefficient/2
  rho/1 -> Dynamic Pressure/2
  Wind-axes Velocities/1 -> VelW/1, Aerodynamic Force/5, Yaw Moment Coefficient/1, Roll Moment Coefficient/1, Pitch Moment Coefficient/1, Side Force Coefficient/1, Drag Coefficient/1, Dynamic Pressure/1, Lift Coefficient/1
  a/1 -> Wind-axes Velocities/3
  WindB/1 -> Wind-axes Velocities/2
  VelB/1 -> Wind-axes Velocities/1

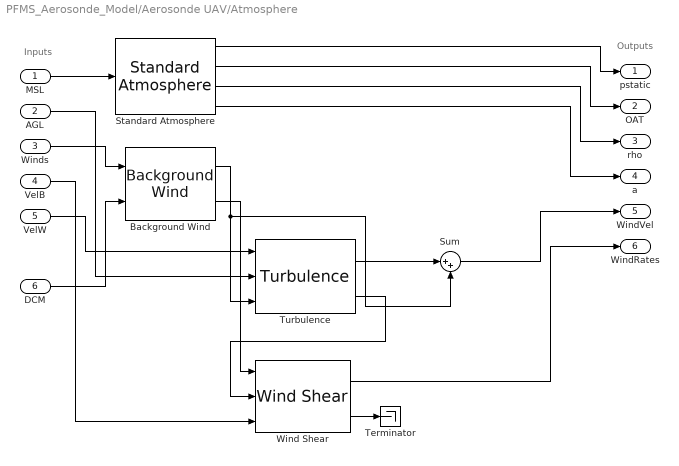
== system PFMS_Aerosonde_Model/Aerosonde UAV/Atmosphere ==
  note: Outputs
  note: Inputs
  MSL : Inport  PortDimensions=1  DataType=double  OutDataType=sfix(16)  OutScaling=2^0  OutDataTypeStr=double
  AGL : Inport  Port=2  PortDimensions=1  DataType=double  OutDataType=sfix(16)  OutScaling=2^0  OutDataTypeStr=double
  Winds : Inport  Port=3  PortDimensions=[3 1]  DataType=double  OutDataType=sfix(16)  OutScaling=2^0  OutDataTypeStr=double
  VelB : Inport  Port=4  PortDimensions=[3 1]  DataType=double  OutDataType=sfix(16)  OutScaling=2^0  OutDataTypeStr=double
  VelW : Inport  Port=5  PortDimensions=[3 1]  OutDataType=sfix(16)  OutScaling=2^0
  DCM : Inport  Port=6  PortDimensions=[3 3]  DataType=double  OutDataType=sfix(16)  OutScaling=2^0  OutDataTypeStr=double
  Background Wind : aerosimlib/Atmosphere/Background Wind  SystemSampleTime=-1
  Standard Atmosphere : aerosimlib/Atmosphere/Standard Atmosphere  SystemSampleTime=-1
  Sum : Sum  Inputs=|++  OutDataType=sfix(16)  OutScaling=2^0  SaturateOnIntegerOverflow=on  InputSameDT=on  OutDataTypeStr=Inherit: Same as first input
  Terminator : Terminator
  Turbulence : aerosimlib/Atmosphere/Turbulence  SystemSampleTime=-1  tsamp=tsamp
  Wind Shear : aerosimlib/Atmosphere/Wind Shear  SystemSampleTime=-1
  pstatic : Outport
  OAT : Outport  Port=2
  rho : Outport  Port=3
  a : Outport  Port=4
  WindVel : Outport  Port=5
  WindRates : Outport  Port=6
  wires:
  Wind Shear/2 -> Terminator/1
  Sum/1 -> WindVel/1
  Standard Atmosphere/4 -> a/1
  Standard Atmosphere/3 -> rho/1
  Standard Atmosphere/2 -> OAT/1
  Standard Atmosphere/1 -> pstatic/1
  Wind Shear/1 -> WindRates/1
  VelB/1 -> Wind Shear/3
  Turbulence/2 -> Wind Shear/2
  Turbulence/1 -> Sum/1
  Background Wind/2 -> Wind Shear/1
  VelW/1 -> Turbulence/1
  AGL/1 -> Turbulence/2
  Background Wind/1 -> Sum/2, Turbulence/3
  DCM/1 -> Background Wind/2
  Winds/1 -> Background Wind/1
  MSL/1 -> Standard Atmosphere/1

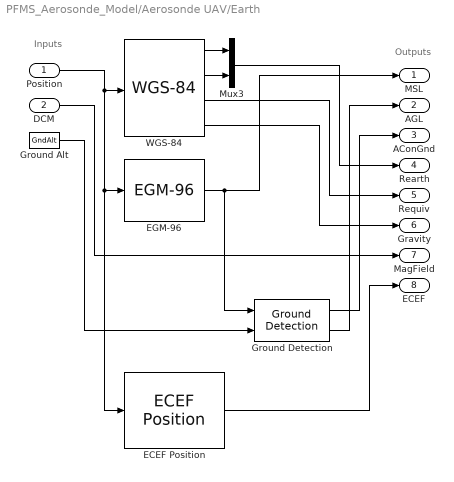
== system PFMS_Aerosonde_Model/Aerosonde UAV/Earth ==
  note: Outputs
  note: Inputs
  Position : Inport  PortDimensions=[3 1]  DataType=double  OutDataType=sfix(16)  OutScaling=2^0  OutDataTypeStr=double
  DCM : Inport  Port=2  PortDimensions=[3 3]  DataType=double  OutDataType=sfix(16)  OutScaling=2^0  OutDataTypeStr=double
  ECEF Position : aerosimlib/Transformations/ECEF Position  SystemSampleTime=-1
  EGM-96 : aerosimlib/Earth/EGM-96  SystemSampleTime=-1
  Ground Alt : Constant  Value=GndAlt  OutDataType=sfix(16)  OutScaling=2^0
  Ground Detection : aerosimlib/Earth/Ground Detection  SystemSampleTime=-1
  Mux3 : Mux  Inputs=2
  WGS-84 : aerosimlib/Earth/WGS-84  SystemSampleTime=-1
  MSL : Outport
  AGL : Outport  Port=2
  AConGnd : Outport  Port=3
  Rearth : Outport  Port=4
  Requiv : Outport  Port=5
  Gravity : Outport  Port=6
  MagField : Outport  Port=7
  ECEF : Outport  Port=8
  wires:
  ECEF Position/1 -> ECEF/1
  WGS-84/4 -> Gravity/1
  WGS-84/3 -> Requiv/1
  Mux3/1 -> Rearth/1
  Ground Detection/1 -> AConGnd/1
  Ground Detection/2 -> AGL/1
  WGS-84/2 -> Mux3/2
  WGS-84/1 -> Mux3/1
  EGM-96/1 -> MSL/1, Ground Detection/1
  Ground Alt/1 -> Ground Detection/2
  Position/1 -> EGM-96/1, ECEF Position/1, WGS-84/1
  DCM/1 -> MagField/1

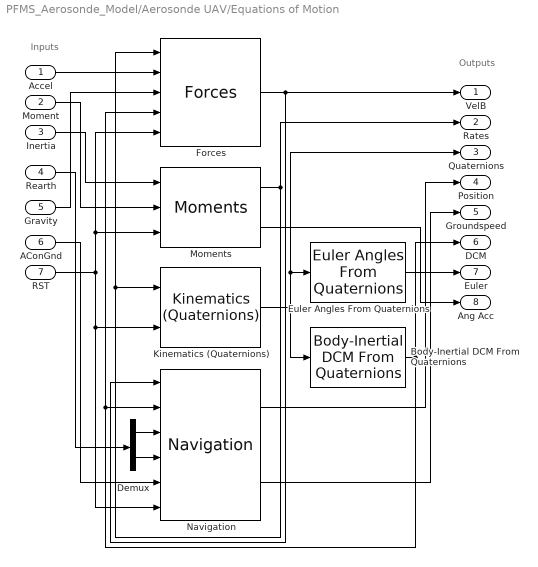
== system PFMS_Aerosonde_Model/Aerosonde UAV/Equations of Motion ==
  note: Inputs
  note: Outputs
  Accel : Inport  PortDimensions=[3 1]  OutDataType=sfix(16)  OutScaling=2^0
  Moment : Inport  Port=2  PortDimensions=[3 1]  OutDataType=sfix(16)  OutScaling=2^0
  Inertia : Inport  Port=3  PortDimensions=[4 1]  OutDataType=sfix(16)  OutScaling=2^0
  Rearth : Inport  Port=4  PortDimensions=[2 1]  OutDataType=sfix(16)  OutScaling=2^0
  Gravity : Inport  Port=5  PortDimensions=1  OutDataType=sfix(16)  OutScaling=2^0
  AConGnd : Inport  Port=6  PortDimensions=1  OutDataType=sfix(16)  OutScaling=2^0
  RST : Inport  Port=7  PortDimensions=1  OutDataType=sfix(16)  OutScaling=2^0
  Body-Inertial DCM From Quaternions : aerosimlib/Transformations/Body-Inertial DCM From Quaternions  SystemSampleTime=-1
  Demux : Demux  Outputs=2
  Euler Angles From Quaternions : aerosimlib/Transformations/Euler Angles From Quaternions  SystemSampleTime=-1
  Forces : aerosimlib/Equations of Motion/Body-Frame EOM/Forces  SystemSampleTime=-1  VelocitiesIni=VelocitiesIni
  Kinematics (Quaternions) : aerosimlib/Equations of Motion/Body-Frame EOM/Kinematics (Quaternions)  SystemSampleTime=-1  QuaternionsIni=QuaternionsIni
  Moments : aerosimlib/Equations of Motion/Body-Frame EOM/Moments  SystemSampleTime=-1  RatesIni=RatesIni
  Navigation : aerosimlib/Equations of Motion/Body-Frame EOM/Navigation  SystemSampleTime=-1  PositionIni=PositionIni
  VelB : Outport
  Rates : Outport  Port=2
  Quaternions : Outport  Port=3
  Position : Outport  Port=4
  Groundspeed : Outport  Port=5
  DCM : Outport  Port=6
  Euler : Outport  Port=7
  Ang Acc : Outport  Port=8
  wires:
  Navigation/2 -> Groundspeed/1
  Navigation/1 -> Position/1
  Moments/2 -> Ang Acc/1
  RST/1 -> Kinematics (Quaternions)/2, Navigation/6, Moments/3, Forces/5
  Moments/1 -> Rates/1, Kinematics (Quaternions)/1, Forces/1
  Kinematics (Quaternions)/1 -> Body-Inertial DCM From Quaternions/1, Euler Angles From Quaternions/1, Quaternions/1
  Forces/1 -> Navigation/1, VelB/1
  AConGnd/1 -> Navigation/5
  Gravity/1 -> Forces/3
  Inertia/1 -> Moments/1
  Moment/1 -> Moments/2
  Accel/1 -> Forces/2
  Demux/2 -> Navigation/4
  Demux/1 -> Navigation/3
  Rearth/1 -> Demux/1
  Body-Inertial DCM From Quaternions/1 -> Navigation/2, Forces/4, DCM/1
  Euler Angles From Quaternions/1 -> Euler/1

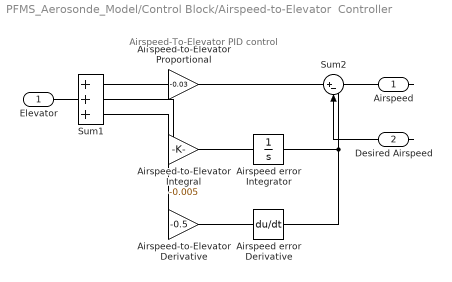
== system PFMS_Aerosonde_Model/Control Block/Airspeed-to-Elevator  Controller ==
  note: Airspeed-To-Elevator PID control
  Airspeed : Inport
  Desired Airspeed : Inport  Port=2
  Airspeed error Derivative : Derivative
  Airspeed error Integrator : Integrator
  Airspeed-to-Elevator Derivative : Gain  Gain=-0.5  SaturateOnIntegerOverflow=on  OutDataTypeStr=Inherit: Same as input  ParamDataTypeStr=Inherit: Same as input
  Airspeed-to-Elevator Integral : Gain  Gain=-0.005  SaturateOnIntegerOverflow=on  OutDataTypeStr=Inherit: Same as input  ParamDataTypeStr=Inherit: Same as input
  Airspeed-to-Elevator Proportional : Gain  Gain=-0.03  SaturateOnIntegerOverflow=on  OutDataTypeStr=Inherit: Same as input  ParamDataTypeStr=Inherit: Same as input
  Sum1 : Sum  Inputs=+++  SaturateOnIntegerOverflow=on  InputSameDT=on  OutDataTypeStr=Inherit: Same as first input
  Sum2 : Sum  Inputs=|+-  SaturateOnIntegerOverflow=on  InputSameDT=on  OutDataTypeStr=Inherit: Same as first input
  Elevator : Outport
  wires:
  Airspeed error Derivative/1 -> Airspeed-to-Elevator Derivative/1
  Airspeed error Integrator/1 -> Airspeed-to-Elevator Integral/1
  Airspeed-to-Elevator Proportional/1 -> Sum1/1
  Airspeed-to-Elevator Integral/1 -> Sum1/2
  Airspeed-to-Elevator Derivative/1 -> Sum1/3
  Sum2/1 -> Airspeed-to-Elevator Proportional/1, Airspeed error Integrator/1, Airspeed error Derivative/1
  Airspeed/1 -> Sum2/1
  Sum1/1 -> Elevator/1
  Desired Airspeed/1 -> Sum2/2

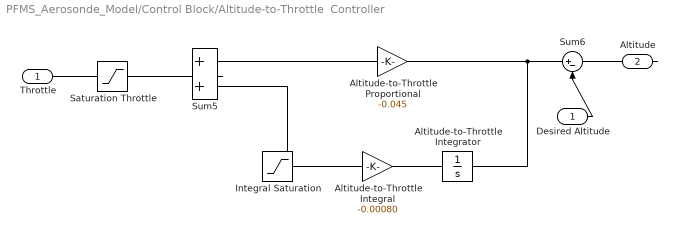
== system PFMS_Aerosonde_Model/Control Block/Altitude-to-Throttle  Controller ==
  Desired Altitude : Inport
  Altitude : Inport  Port=2
  Altitude-to-Throttle Integral : Gain  Gain=-0.00080  SaturateOnIntegerOverflow=on  OutDataTypeStr=Inherit: Same as input  ParamDataTypeStr=Inherit: Same as input
  Altitude-to-Throttle Integrator : Integrator
  Altitude-to-Throttle Proportional : Gain  Gain=-0.045  SaturateOnIntegerOverflow=on  OutDataTypeStr=Inherit: Same as input  ParamDataTypeStr=Inherit: Same as input
  Integral Saturation : Saturate  UpperLimit=.8  LowerLimit=0  OutDataType=fixdt(1, 16)  OutScaling=2^0
  Saturation Throttle : Saturate  UpperLimit=1.5  LowerLimit=0  OutDataType=fixdt(1, 16)  OutScaling=2^0
  Sum5 : Sum  SaturateOnIntegerOverflow=on  InputSameDT=on  OutDataTypeStr=Inherit: Same as first input
  Sum6 : Sum  Inputs=|+-  OutDataType=fixdt(1, 16)  OutScaling=2^0
  Throttle : Outport
  wires:
  Sum6/1 -> Altitude-to-Throttle Proportional/1, Altitude-to-Throttle Integrator/1
  Integral Saturation/1 -> Sum5/2
  Altitude-to-Throttle Integral/1 -> Integral Saturation/1
  Sum5/1 -> Saturation Throttle/1
  Altitude-to-Throttle Proportional/1 -> Sum5/1
  Altitude-to-Throttle Integrator/1 -> Altitude-to-Throttle Integral/1
  Altitude/1 -> Sum6/1
  Desired Altitude/1 -> Sum6/2
  Saturation Throttle/1 -> Throttle/1

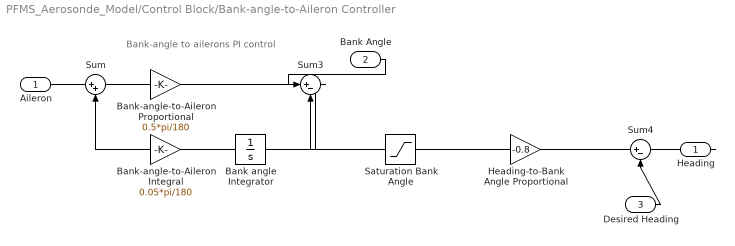
== system PFMS_Aerosonde_Model/Control Block/Bank-angle-to-Aileron Controller ==
  note: Bank-angle to ailerons PI control
  Heading : Inport
  Bank Angle : Inport  Port=2
  Desired Heading : Inport  Port=3
  Bank angle Integrator : Integrator
  Bank-angle-to-Aileron Integral : Gain  Gain=0.05*pi/180  SaturateOnIntegerOverflow=on  OutDataTypeStr=Inherit: Same as input  ParamDataTypeStr=Inherit: Same as input
  Bank-angle-to-Aileron Proportional : Gain  Gain=0.5*pi/180  SaturateOnIntegerOverflow=on  OutDataTypeStr=Inherit: Same as input  ParamDataTypeStr=Inherit: Same as input
  Heading-to-Bank Angle Proportional : Gain  Gain=-0.8  SaturateOnIntegerOverflow=on  OutDataTypeStr=Inherit: Same as input  ParamDataTypeStr=Inherit: Same as input
  Saturation Bank Angle : Saturate  UpperLimit=20  LowerLimit=-20  OutDataType=fixdt(1, 16)  OutScaling=2^0
  Sum : Sum  Inputs=|++  SaturateOnIntegerOverflow=on  InputSameDT=on  OutDataTypeStr=Inherit: Same as first input
  Sum3 : Sum  Inputs=|+-  SaturateOnIntegerOverflow=on  InputSameDT=on  OutDataTypeStr=Inherit: Same as first input
  Sum4 : Sum  Inputs=|+-  OutDataType=fixdt(1, 16)  OutScaling=2^0
  Aileron : Outport
  wires:
  Sum3/1 -> Bank-angle-to-Aileron Proportional/1, Bank angle Integrator/1
  Bank-angle-to-Aileron Integral/1 -> Sum/2
  Bank angle Integrator/1 -> Bank-angle-to-Aileron Integral/1
  Bank-angle-to-Aileron Proportional/1 -> Sum/1
  Sum4/1 -> Heading-to-Bank Angle Proportional/1
  Heading-to-Bank Angle Proportional/1 -> Saturation Bank Angle/1
  Heading/1 -> Sum4/1
  Bank Angle/1 -> Sum3/1
  Desired Heading/1 -> Sum4/2
  Sum/1 -> Aileron/1
  Saturation Bank Angle/1 -> Sum3/2
